simulink model "Ver1"  (R2025a)
settings: Solver=VariableStepAuto  StartTime=0.0  StopTime=50  RelTol=1e-3
model workspace (MAT data in the model file):
  params = Simulink.Parameter
  params.Value.graph_params.n_drones = 10
  params.Value.graph_params.n_vertex = 10
  params.Value.graph_params.dim = 3
  params.Value.graph_params.edges = [1  2; 1  3; 1  4; 1  5; 1  6; 1  7; 1  8; 1  9; 1  10; 2  3; 3  4; 4  5; 5  6; 6  7; 7  8; 8  9; 9  10; 10  2; 2  4; 3  5; 4  6; 5  7; 6  8; 7  9; 8  10; 9  2; 2  5; 3  6; 4  7; 5  8; 6  9; 7  10; 8  2; 9  3; 2  7; 3  8; 4  9; 5  10]
  params.Value.leader_params.gamma_leader = 5
  params.Value.leader_params.beta_leader = 20
  params.Value.formation_params.alpha = 0.1
  params.Value.formation_params.beta = 5
  params.Value.formation_params.kp = 0.1
  params.Value.formation_params.kd = 0.2
  params.Value.formation_params.d_star = [12; 12.3583419921; 12.0437867802; 12.2780291578; 12.153953398; 12.153953398; 12.2780291578; 12.0437867802; 12.3583419921; 8.7239794346; 8.43195016483; 8.97293523752; 8.23575839836; 9.06937336224; 8.23575839836; 8.97293523752; 8.43195016483; 8.7239794346; 15.4609871883; 16.3957181972; 15.70725761; 16.0772502381; 16.0772502381; 15.70725761; 16.3957181972; 15.4609871883; 20.9463600657; 21.3504473017; 20.8041858677; 21.4242852856; 20.8041858677; 21.3504473017; 20.9463600657; 21.1623309302; 23.7139211854; 23.6380722142; 23.7243055707; 23.6380722142]
  params.Value.avoid_params.k = 0.3
  params.Value.avoid_params.alpha = 2
  params.Value.avoid_params.d_safe = 5
  params.Value.conn_params.omega = 30
  params.Value.conn_params.alpha = 4
  params.Value.conn_params.d_max = 100
  params.Value.conn_params.Q = [-0.504121366584  -0.26105915892  -0.171736950093  -0.315040358305  -0.405829965319  0.0998199433836  -0.438792761923  -0.20112384887  0.203258169728; 0.156957729109  -0.265892972159  -0.546045591004  0.250622322861  0.326889653272  0.0848989604996  -0.256821652418  -0.050927060205  -0.510952303973; -0.317453653204  -0.3194315981  0.431976209598  -0.0284937114609  0.594225330731  -0.201716490834  0.193668666917  -0.272418527482  0.0652579645217; -0.13048124049  -0.134179261876  0.122212763196  -0.0870348158074  -0.0371148175386  -0.151496335719  0.0161251708109  0.899410389048  -0.0945083828758; 0.192528892253  -0.114548534632  0.205433346657  -0.218675435515  -0.474708640435  0.0269386697665  0.459932147337  -0.227364089546  -0.52008024212; 0.369488953482  0.322391236465  0.52165561704  -0.0285219597056  0.0532846827894  0.159326821637  -0.592803250035  -0.0504485144303  -0.0664731491506; -0.415313062767  0.706628196345  -0.139244596418  0.283837891368  -0.0540882463489  -0.300425585948  0.0949860236049  -0.0883544592836  -0.135013775508; 0.450114303089  0.121748450665  -0.342077032843  -0.467416117234  0.120960097676  -0.427451020909  0.0961435138919  -0.0562630144241  0.370573991674; 0.231595539246  -0.260589900824  0.050268923297  0.689669598678  -0.307348035599  -0.0738893443802  0.0890571931834  -0.0373520916293  0.437077198207; -0.033316094133  0.204933543037  -0.132442689429  -0.0789474148786  0.183729940772  0.783994382503  0.338504948631  0.0848412168229  0.250860529497]
  params.Value.estimation_params.mu = 1.2
  params.Value.prior_params.k_form = 5
  params.Value.prior_params.k_back = 1
  params.Value.prior_params.k_damp = 1
  params.Value.prior_params.k_conn = 0.5
  params.Value.prior_params.k_avoid = 10
  params.Value.prior_params.k_height = 25
  params.Complexity = 'real'
  params.Dimensions = [1 1]
  params.DataType = 'Bus: slBus8'
values from neighbouring files (symbols this model uses):
  edges = getappdata(0, 'DataEdges')    [DataAnalysis.m]    (also in Data_Analysis.m = graph_params.edges; Trajectory.m = getappdata(0, 'Edges'); data.m = graph_params.edges; formation_data.mat = [1 1 1 1 1 1 1 1 1 1 2 3 ... (62 elements, 31x2)])
  p10_init = [9; 5; 0]    [data.m]
  p2_init = [10; 0; 0]    [data.m]
  p3_init = [0; 10; 0]    [data.m]
  p4_init = [-10; 0; 0]    [data.m]
  p5_init = [0; -10; 0]    [data.m]
  p6_init = [7; 7; 0]    [data.m]
  p7_init = [-7; 7; 0]    [data.m]
  p8_init = [-7; -7; 0]    [data.m]
  p9_init = [7; -7; 0]    [data.m]
(part 1 of 3)
settings Model: Creator=huy01  LastModifiedBy=huy01

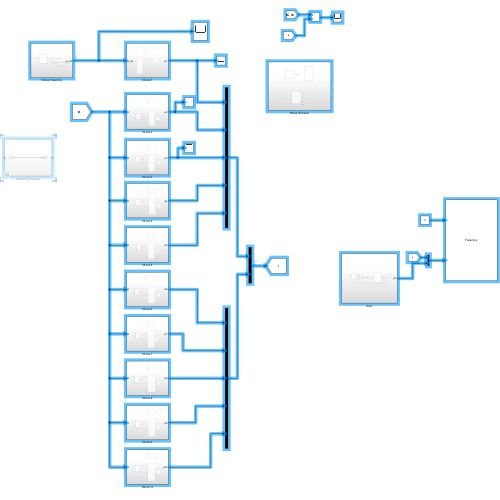
[thumbnail: Simulink's stored preview of the top-level diagram]
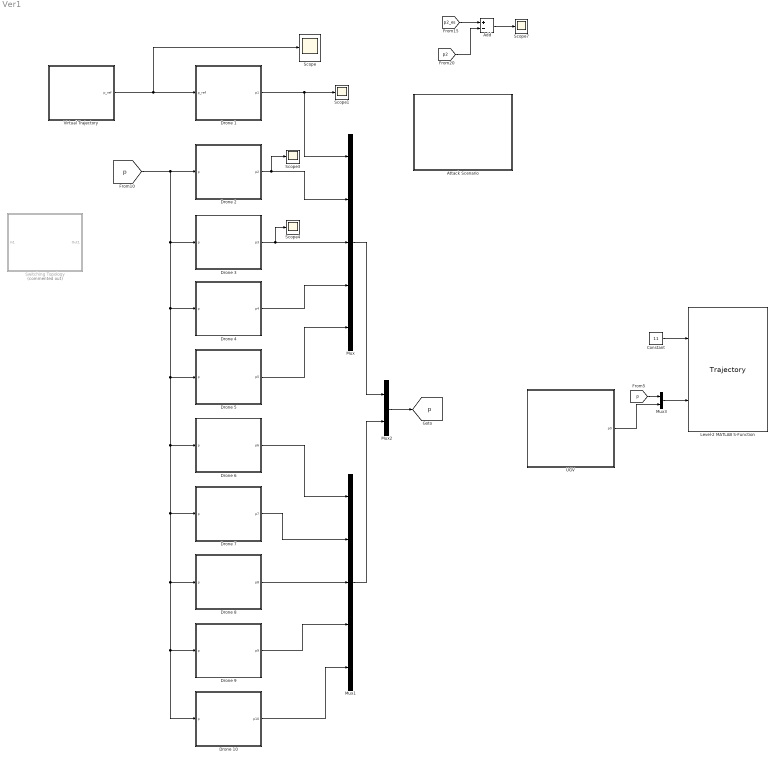
== system Ver1 ==
  Add : Sum  Inputs=+-
  Attack Scenario : Subsystem
  Constant : Constant  Value=11
  Drone 1 : Subsystem
  Drone 10 : Subsystem
  Drone 2 : Subsystem
  Drone 3 : Subsystem
  Drone 4 : Subsystem
  Drone 5 : Subsystem
  Drone 6 : Subsystem
  Drone 7 : Subsystem
  Drone 8 : Subsystem
  Drone 9 : Subsystem
  Level-2 MATLAB S-Function : M-S-Function  FunctionName=Trajectory
  Mux : Mux  Inputs=5
  Mux1 : Mux  Inputs=5
  Mux2 : Mux  Inputs=2
  Mux3 : Mux  Inputs=2
  Scope{,1,3..4,7} (5 alike) : Scope
      Scope settings: ActiveDisplayYMinimum=-6.2499999999999982  ActiveDisplayYMaximum=56.25
      Scope1 settings: ActiveDisplayYMinimum=-3.1816184672991272  ActiveDisplayYMaximum=28.634566205692153
      Scope3 settings: ActiveDisplayYMinimum=-20.171264012877725  ActiveDisplayYMaximum=51.444926631069329  DataLoggingVariableName=ScopeData3
      Scope4 settings: ActiveDisplayYMinimum=-35.468264300452987  ActiveDisplayYMaximum=33.637957066493193  DataLoggingVariableName=ScopeData4
      Scope7 settings: ActiveDisplayYMinimum=-11.251507111001377  ActiveDisplayYMaximum=1.2635639990123921  DataLoggingVariableName=ScopeData10
  Switching Topology : Subsystem  Commented=on
  UGV : Subsystem
  Virtual Trajectory : Subsystem
  tag scope: p=global
  wires:
  UGV/1(p0) -> Mux3/2
  [p2] -> Add/2
  Mux/1 -> Mux2/1
  Drone 10/1(p10) -> Mux1/5
  Mux3/1 -> Level-2 MATLAB S-Function/2
  [p] -> Mux3/1
  Drone 1/1(p1) -> Mux/1, Scope1/1
  [p2_es] -> Add/1
  [p] -> Drone 5/1(p), Drone 10/1(p), Drone 9/1(p), Drone 8/1(p), Drone 7/1(p), Drone 6/1(p), Drone 4/1(p), Drone 3/1(p), Drone 2/1(p)
  Add/1 -> Scope7/1
  Mux1/1 -> Mux2/2
  Drone 2/1(p2) -> Scope3/1, Mux/2
  Drone 9/1(p9) -> Mux1/4
  Drone 6/1(p6) -> Mux1/1
  Drone 5/1(p5) -> Mux/5
  Constant/1 -> Level-2 MATLAB S-Function/1
  Mux2/1 -> [p]
  Drone 4/1(p4) -> Mux/4
  Drone 7/1(p7) -> Mux1/2
  Drone 3/1(p3) -> Scope4/1, Mux/3
  Drone 8/1(p8) -> Mux1/3
  Virtual Trajectory/1(p_ref) -> Scope/1, Drone 1/1(p_ref)

== system Ver1/Attack Scenario ==
  Attacker : MATLAB Function  Commented=on  TreatAsAtomicUnit=on
  Data : Subsystem
  MATLAB Function : MATLAB Function  TreatAsAtomicUnit=on
  Scope : Scope
      settings: ActiveDisplayYMinimum=-20.35285300251708  ActiveDisplayYMaximum=217.26420858699828  DataLoggingVariableName=ScopeData2
  Scope1 : Scope
      settings: ActiveDisplayYMinimum=3.25  ActiveDisplayYMaximum=10.75  DataLoggingVariableName=ScopeData5
  Scope2 : Scope
      settings: ActiveDisplayYMinimum=-1.2499999999999998  ActiveDisplayYMaximum=11.25  DataLoggingVariableName=ScopeData6
  tag scope: n=global, p_es=global
  wires:
  Data/1(pes) -> [p_es]
  [p] -> MATLAB Function/1(p)
  [p0] -> MATLAB Function/2(p0)
  MATLAB Function/1(d1) -> Scope/1
  MATLAB Function/2(i_min) -> Scope1/1
  MATLAB Function/3(n) -> [n], Scope2/1

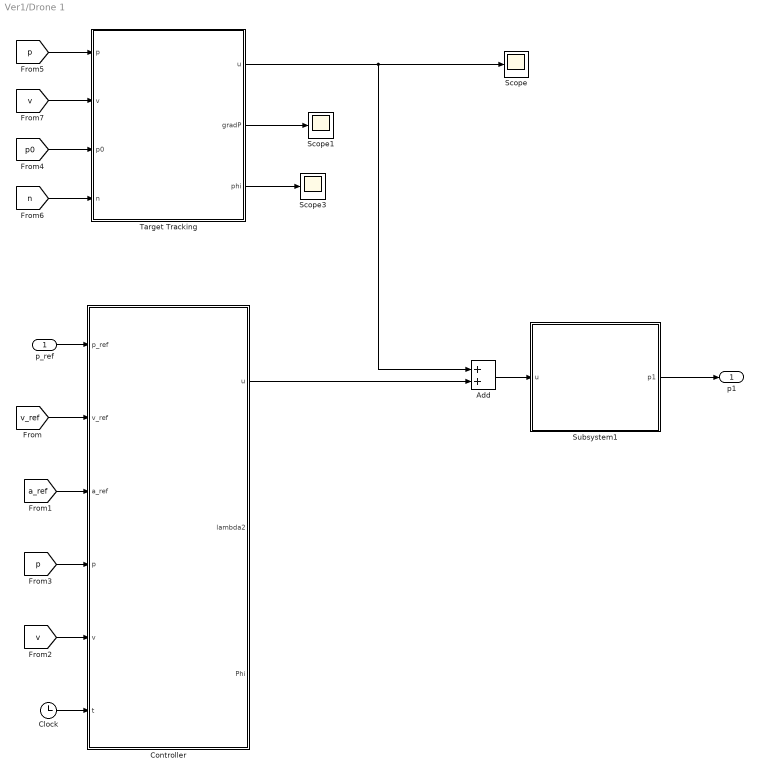
== system Ver1/Drone 1 ==
  p_ref : Inport
  Add : Sum
  Clock : Clock
  Controller : MATLAB Function  TreatAsAtomicUnit=on
  Scope : Scope
      settings: ActiveDisplayYMinimum=-25  ActiveDisplayYMaximum=25  DataLoggingVariableName=ScopeData17
  Scope1 : Scope
      settings: ActiveDisplayYMinimum=-1  ActiveDisplayYMaximum=1  DataLoggingVariableName=ScopeData18
  Scope3 : Scope
      settings: ActiveDisplayYMinimum=-1.1694156754654319E+234  ActiveDisplayYMaximum=1.0524741079188889E+235  DataLoggingVariableName=ScopeData20
  Subsystem1 : Subsystem
  Target Tracking : MATLAB Function  TreatAsAtomicUnit=on
  p1 : Outport
  wires:
  [v] -> Controller/5(v)
  [p] -> Controller/4(p)
  Subsystem1/1(p1) -> p1/1
  [p0] -> Target Tracking/3(p0)
  [p] -> Target Tracking/1(p)
  Target Tracking/1(u) -> Scope/1, Add/1
  [n] -> Target Tracking/4(n)
  Target Tracking/2(gradP) -> Scope1/1
  [v] -> Target Tracking/2(v)
  Target Tracking/3(phi) -> Scope3/1
  Add/1 -> Subsystem1/1(u)
  Controller/1(u) -> Add/2
  p_ref/1 -> Controller/1(p_ref)
  [a_ref] -> Controller/3(a_ref)
  Clock/1 -> Controller/6(t)
  [v_ref] -> Controller/2(v_ref)

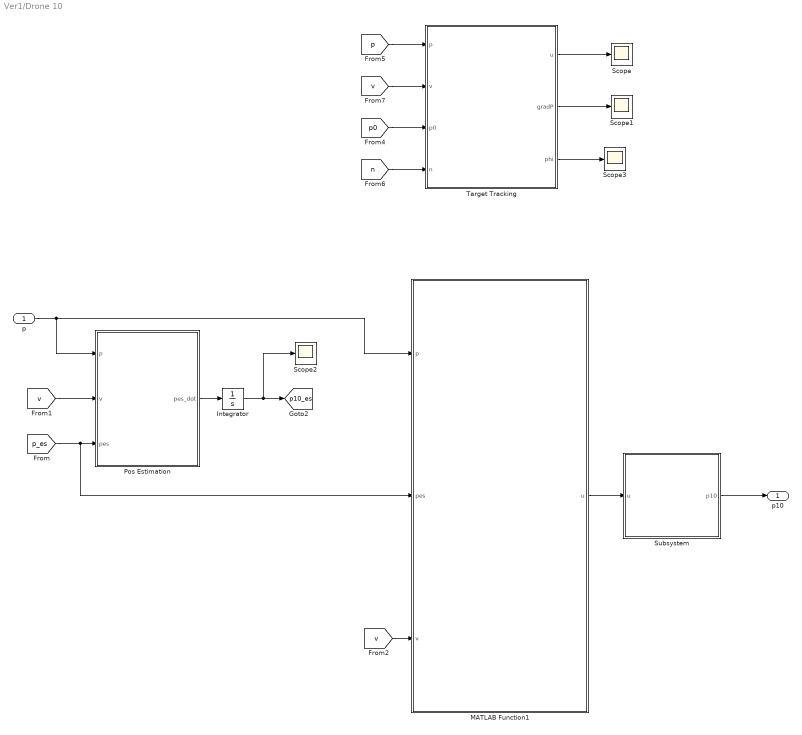
== system Ver1/Drone 10 ==
  p : Inport
  Integrator : Integrator  InitialCondition=[0;0;0]
  MATLAB Function1 : MATLAB Function  TreatAsAtomicUnit=on
  Pos Estimation : MATLAB Function  TreatAsAtomicUnit=on
  Scope{,1..3} (4 alike) : Scope
      Scope settings: ActiveDisplayYMinimum=-25  ActiveDisplayYMaximum=25  DataLoggingVariableName=ScopeData44
      Scope1 settings: ActiveDisplayYMinimum=-1  ActiveDisplayYMaximum=1  DataLoggingVariableName=ScopeData45
      Scope2 settings: DataLoggingVariableName=ScopeData13
      Scope3 settings: ActiveDisplayYMinimum=-1.1694156754654319E+234  ActiveDisplayYMaximum=1.0524741079188889E+235  DataLoggingVariableName=ScopeData46
  Subsystem : Subsystem
  Target Tracking : MATLAB Function  TreatAsAtomicUnit=on
  p10 : Outport
  tag scope: p10_es=global
  wires:
  Subsystem/1(p10) -> p10/1
  [v] -> MATLAB Function1/3(v)
  Integrator/1 -> Scope2/1, [p10_es]
  p/1 -> Pos Estimation/1(p), MATLAB Function1/1(p)
  Pos Estimation/1(pes_dot) -> Integrator/1
  [p_es] -> MATLAB Function1/2(pes), Pos Estimation/3(pes)
  [v] -> Target Tracking/2(v)
  Target Tracking/3(phi) -> Scope3/1
  [p0] -> Target Tracking/3(p0)
  Target Tracking/2(gradP) -> Scope1/1
  [n] -> Target Tracking/4(n)
  Target Tracking/1(u) -> Scope/1
  [p] -> Target Tracking/1(p)
  MATLAB Function1/1(u) -> Subsystem/1(u)
  [v] -> Pos Estimation/2(v)

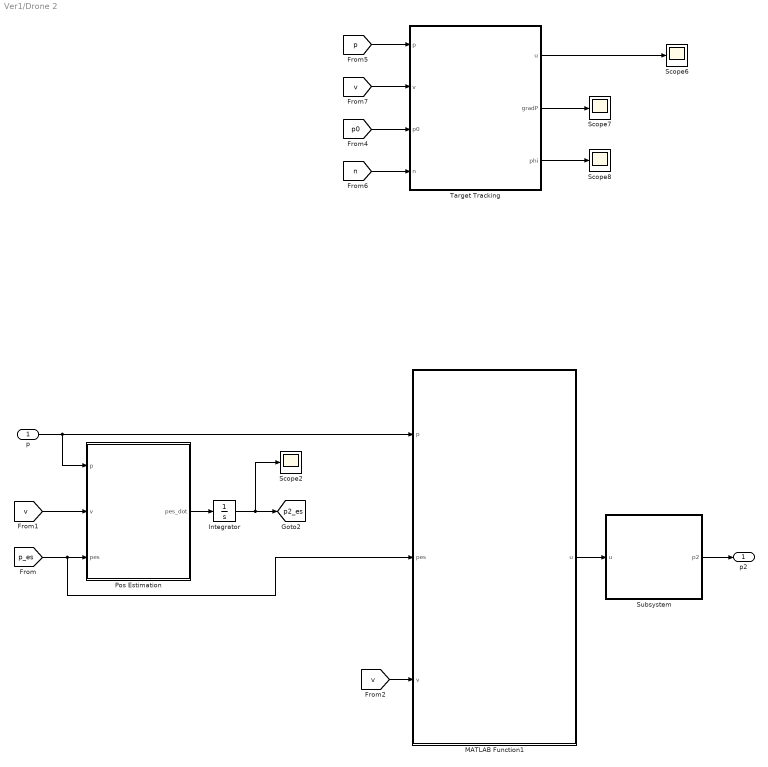
== system Ver1/Drone 2 ==
  p : Inport
  Integrator : Integrator  InitialCondition=[0;0;0]
  MATLAB Function1 : MATLAB Function  TreatAsAtomicUnit=on
  Pos Estimation : MATLAB Function  TreatAsAtomicUnit=on
  Scope{2,6..8} (4 alike) : Scope
      Scope2 settings: ActiveDisplayYMinimum=-1  ActiveDisplayYMaximum=1  DataLoggingVariableName=ScopeData9
      Scope6 settings: ActiveDisplayYMinimum=-25  ActiveDisplayYMaximum=25  DataLoggingVariableName=ScopeData19
      Scope7 settings: ActiveDisplayYMinimum=-1  ActiveDisplayYMaximum=1  DataLoggingVariableName=ScopeData21
      Scope8 settings: ActiveDisplayYMinimum=-1.1694156754654319E+234  ActiveDisplayYMaximum=1.0524741079188889E+235  DataLoggingVariableName=ScopeData22
  Subsystem : Subsystem
  Target Tracking : MATLAB Function  TreatAsAtomicUnit=on
  p2 : Outport
  tag scope: p2_es=global
  wires:
  [v] -> MATLAB Function1/3(v)
  p/1 -> Pos Estimation/1(p), MATLAB Function1/1(p)
  Subsystem/1(p2) -> p2/1
  Pos Estimation/1(pes_dot) -> Integrator/1
  Integrator/1 -> Scope2/1, [p2_es]
  [p_es] -> MATLAB Function1/2(pes), Pos Estimation/3(pes)
  [v] -> Target Tracking/2(v)
  Target Tracking/3(phi) -> Scope8/1
  [p0] -> Target Tracking/3(p0)
  Target Tracking/2(gradP) -> Scope7/1
  [n] -> Target Tracking/4(n)
  Target Tracking/1(u) -> Scope6/1
  [p] -> Target Tracking/1(p)
  MATLAB Function1/1(u) -> Subsystem/1(u)
  [v] -> Pos Estimation/2(v)

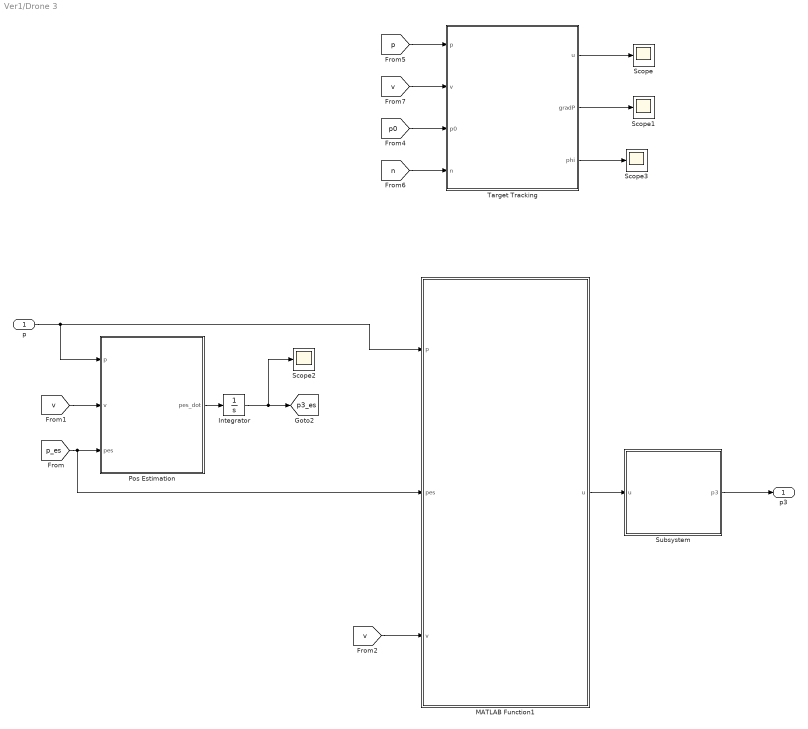
== system Ver1/Drone 3 ==
  p : Inport
  Integrator : Integrator  InitialCondition=[0;0;0]
  MATLAB Function1 : MATLAB Function  TreatAsAtomicUnit=on
  Pos Estimation : MATLAB Function  TreatAsAtomicUnit=on
  Scope{,1..3} (4 alike) : Scope
      Scope settings: ActiveDisplayYMinimum=-25  ActiveDisplayYMaximum=25  DataLoggingVariableName=ScopeData23
      Scope1 settings: ActiveDisplayYMinimum=-1  ActiveDisplayYMaximum=1  DataLoggingVariableName=ScopeData24
      Scope2 settings: ActiveDisplayYMinimum=-1  ActiveDisplayYMaximum=1  DataLoggingVariableName=ScopeData11
      Scope3 settings: ActiveDisplayYMinimum=-1.1694156754654319E+234  ActiveDisplayYMaximum=1.0524741079188889E+235  DataLoggingVariableName=ScopeData25
  Subsystem : Subsystem
  Target Tracking : MATLAB Function  TreatAsAtomicUnit=on
  p3 : Outport
  tag scope: p3_es=global
  wires:
  Subsystem/1(p3) -> p3/1
  [v] -> MATLAB Function1/3(v)
  Integrator/1 -> Scope2/1, [p3_es]
  p/1 -> Pos Estimation/1(p), MATLAB Function1/1(p)
  Pos Estimation/1(pes_dot) -> Integrator/1
  [p_es] -> MATLAB Function1/2(pes), Pos Estimation/3(pes)
  [v] -> Target Tracking/2(v)
  Target Tracking/3(phi) -> Scope3/1
  [p0] -> Target Tracking/3(p0)
  Target Tracking/2(gradP) -> Scope1/1
  [n] -> Target Tracking/4(n)
  Target Tracking/1(u) -> Scope/1
  [p] -> Target Tracking/1(p)
  MATLAB Function1/1(u) -> Subsystem/1(u)
  [v] -> Pos Estimation/2(v)

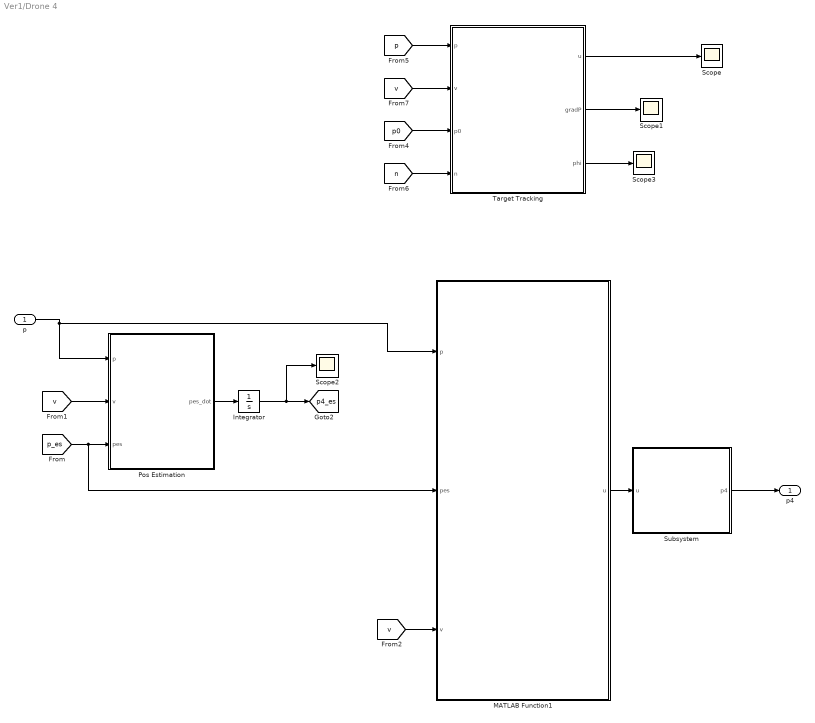
== system Ver1/Drone 4 ==
  p : Inport
  Integrator : Integrator  InitialCondition=[0;0;0]
  MATLAB Function1 : MATLAB Function  TreatAsAtomicUnit=on
  Pos Estimation : MATLAB Function  TreatAsAtomicUnit=on
  Scope{,1..3} (4 alike) : Scope
      Scope settings: ActiveDisplayYMinimum=-25  ActiveDisplayYMaximum=25  DataLoggingVariableName=ScopeData26
      Scope1 settings: ActiveDisplayYMinimum=-1  ActiveDisplayYMaximum=1  DataLoggingVariableName=ScopeData27
      Scope2 settings: DataLoggingVariableName=ScopeData12
      Scope3 settings: ActiveDisplayYMinimum=-1.1694156754654319E+234  ActiveDisplayYMaximum=1.0524741079188889E+235  DataLoggingVariableName=ScopeData28
  Subsystem : Subsystem
  Target Tracking : MATLAB Function  TreatAsAtomicUnit=on
  p4 : Outport
  tag scope: p4_es=global
  wires:
  Subsystem/1(p4) -> p4/1
  [v] -> MATLAB Function1/3(v)
  Integrator/1 -> Scope2/1, [p4_es]
  p/1 -> Pos Estimation/1(p), MATLAB Function1/1(p)
  Pos Estimation/1(pes_dot) -> Integrator/1
  [p_es] -> MATLAB Function1/2(pes), Pos Estimation/3(pes)
  [v] -> Target Tracking/2(v)
  Target Tracking/3(phi) -> Scope3/1
  [p0] -> Target Tracking/3(p0)
  Target Tracking/2(gradP) -> Scope1/1
  [n] -> Target Tracking/4(n)
  Target Tracking/1(u) -> Scope/1
  [p] -> Target Tracking/1(p)
  MATLAB Function1/1(u) -> Subsystem/1(u)
  [v] -> Pos Estimation/2(v)

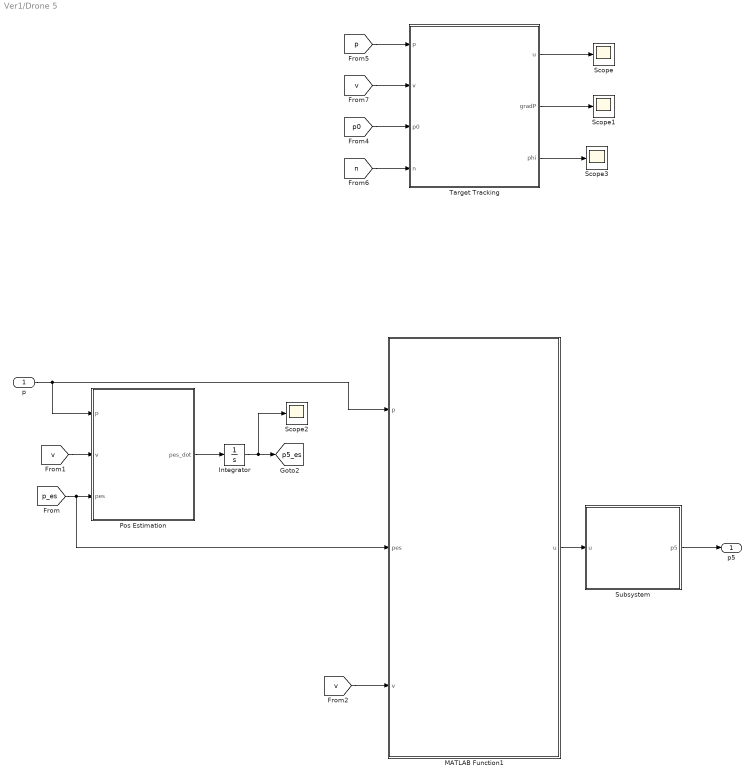
== system Ver1/Drone 5 ==
  p : Inport
  Integrator : Integrator  InitialCondition=[0;0;0]
  MATLAB Function1 : MATLAB Function  TreatAsAtomicUnit=on
  Pos Estimation : MATLAB Function  TreatAsAtomicUnit=on
  Scope{,1..3} (4 alike) : Scope
      Scope settings: ActiveDisplayYMinimum=-25  ActiveDisplayYMaximum=25  DataLoggingVariableName=ScopeData29
      Scope1 settings: ActiveDisplayYMinimum=-1  ActiveDisplayYMaximum=1  DataLoggingVariableName=ScopeData30
      Scope2 settings: DataLoggingVariableName=ScopeData13
      Scope3 settings: ActiveDisplayYMinimum=-1.1694156754654319E+234  ActiveDisplayYMaximum=1.0524741079188889E+235  DataLoggingVariableName=ScopeData31
  Subsystem : Subsystem
  Target Tracking : MATLAB Function  TreatAsAtomicUnit=on
  p5 : Outport
  tag scope: p5_es=global
  wires:
  Subsystem/1(p5) -> p5/1
  [v] -> MATLAB Function1/3(v)
  Integrator/1 -> Scope2/1, [p5_es]
  p/1 -> Pos Estimation/1(p), MATLAB Function1/1(p)
  Pos Estimation/1(pes_dot) -> Integrator/1
  [p_es] -> MATLAB Function1/2(pes), Pos Estimation/3(pes)
  [v] -> Target Tracking/2(v)
  Target Tracking/3(phi) -> Scope3/1
  [p0] -> Target Tracking/3(p0)
  Target Tracking/2(gradP) -> Scope1/1
  [n] -> Target Tracking/4(n)
  Target Tracking/1(u) -> Scope/1
  [p] -> Target Tracking/1(p)
  MATLAB Function1/1(u) -> Subsystem/1(u)
  [v] -> Pos Estimation/2(v)
  ? -> ?

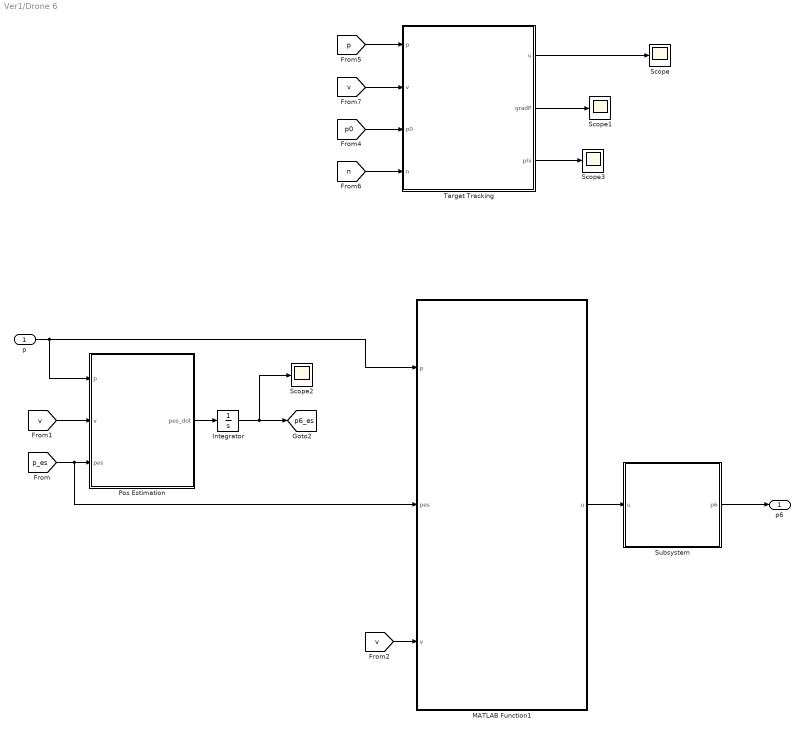
== system Ver1/Drone 6 ==
  p : Inport
  Integrator : Integrator  InitialCondition=[0;0;0]
  MATLAB Function1 : MATLAB Function  TreatAsAtomicUnit=on
  Pos Estimation : MATLAB Function  TreatAsAtomicUnit=on
  Scope{,1..3} (4 alike) : Scope
      Scope settings: ActiveDisplayYMinimum=-25  ActiveDisplayYMaximum=25  DataLoggingVariableName=ScopeData32
      Scope1 settings: ActiveDisplayYMinimum=-1  ActiveDisplayYMaximum=1  DataLoggingVariableName=ScopeData33
      Scope2 settings: DataLoggingVariableName=ScopeData13
      Scope3 settings: ActiveDisplayYMinimum=-1.1694156754654319E+234  ActiveDisplayYMaximum=1.0524741079188889E+235  DataLoggingVariableName=ScopeData34
  Subsystem : Subsystem
  Target Tracking : MATLAB Function  TreatAsAtomicUnit=on
  p6 : Outport
  tag scope: p6_es=global
  wires:
  Subsystem/1(p6) -> p6/1
  [v] -> MATLAB Function1/3(v)
  Integrator/1 -> Scope2/1, [p6_es]
  p/1 -> Pos Estimation/1(p), MATLAB Function1/1(p)
  Pos Estimation/1(pes_dot) -> Integrator/1
  [p_es] -> MATLAB Function1/2(pes), Pos Estimation/3(pes)
  [v] -> Target Tracking/2(v)
  Target Tracking/3(phi) -> Scope3/1
  [p0] -> Target Tracking/3(p0)
  Target Tracking/2(gradP) -> Scope1/1
  [n] -> Target Tracking/4(n)
  Target Tracking/1(u) -> Scope/1
  [p] -> Target Tracking/1(p)
  MATLAB Function1/1(u) -> Subsystem/1(u)
  [v] -> Pos Estimation/2(v)

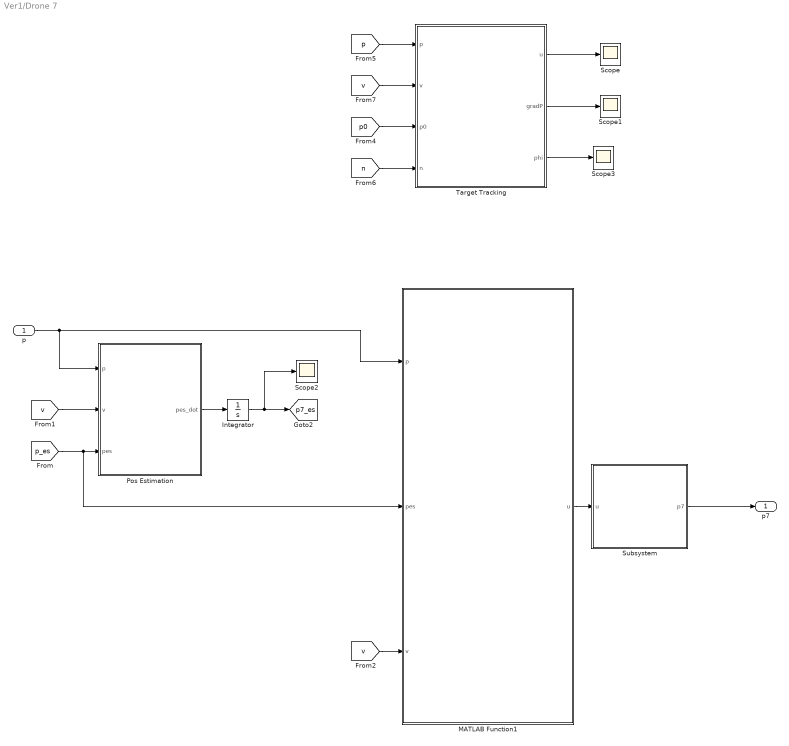
== system Ver1/Drone 7 ==
  p : Inport
  Integrator : Integrator  InitialCondition=[0;0;0]
  MATLAB Function1 : MATLAB Function  TreatAsAtomicUnit=on
  Pos Estimation : MATLAB Function  TreatAsAtomicUnit=on
  Scope{,1..3} (4 alike) : Scope
      Scope settings: ActiveDisplayYMinimum=-25  ActiveDisplayYMaximum=25  DataLoggingVariableName=ScopeData35
      Scope1 settings: ActiveDisplayYMinimum=-1  ActiveDisplayYMaximum=1  DataLoggingVariableName=ScopeData36
      Scope2 settings: DataLoggingVariableName=ScopeData13
      Scope3 settings: ActiveDisplayYMinimum=-1.1694156754654319E+234  ActiveDisplayYMaximum=1.0524741079188889E+235  DataLoggingVariableName=ScopeData37
  Subsystem : Subsystem
  Target Tracking : MATLAB Function  TreatAsAtomicUnit=on
  p7 : Outport
  tag scope: p7_es=global
  wires:
  Subsystem/1(p7) -> p7/1
  [v] -> MATLAB Function1/3(v)
  Integrator/1 -> Scope2/1, [p7_es]
  p/1 -> Pos Estimation/1(p), MATLAB Function1/1(p)
  Pos Estimation/1(pes_dot) -> Integrator/1
  [p_es] -> MATLAB Function1/2(pes), Pos Estimation/3(pes)
  [v] -> Target Tracking/2(v)
  Target Tracking/3(phi) -> Scope3/1
  [p0] -> Target Tracking/3(p0)
  Target Tracking/2(gradP) -> Scope1/1
  [n] -> Target Tracking/4(n)
  Target Tracking/1(u) -> Scope/1
  [p] -> Target Tracking/1(p)
  MATLAB Function1/1(u) -> Subsystem/1(u)
  [v] -> Pos Estimation/2(v)

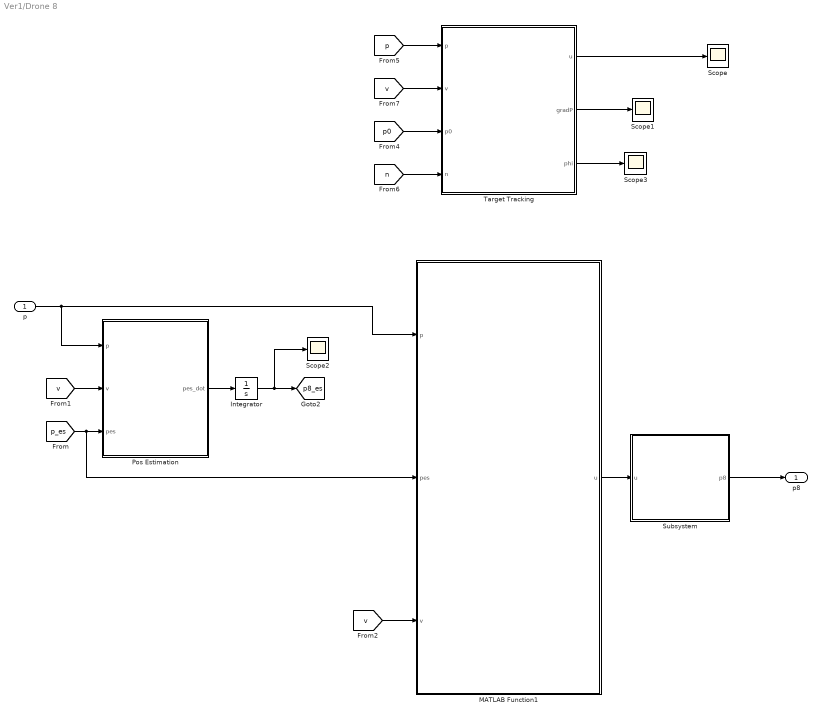
== system Ver1/Drone 8 ==
  p : Inport
  Integrator : Integrator  InitialCondition=[0;0;0]
  MATLAB Function1 : MATLAB Function  TreatAsAtomicUnit=on
  Pos Estimation : MATLAB Function  TreatAsAtomicUnit=on
  Scope{,1..3} (4 alike) : Scope
      Scope settings: ActiveDisplayYMinimum=-25  ActiveDisplayYMaximum=25  DataLoggingVariableName=ScopeData38
      Scope1 settings: ActiveDisplayYMinimum=-1  ActiveDisplayYMaximum=1  DataLoggingVariableName=ScopeData39
      Scope2 settings: DataLoggingVariableName=ScopeData13
      Scope3 settings: ActiveDisplayYMinimum=-1.1694156754654319E+234  ActiveDisplayYMaximum=1.0524741079188889E+235  DataLoggingVariableName=ScopeData40
  Subsystem : Subsystem
  Target Tracking : MATLAB Function  TreatAsAtomicUnit=on
  p8 : Outport
  tag scope: p8_es=global
  wires:
  Subsystem/1(p8) -> p8/1
  [v] -> MATLAB Function1/3(v)
  Integrator/1 -> Scope2/1, [p8_es]
  p/1 -> Pos Estimation/1(p), MATLAB Function1/1(p)
  Pos Estimation/1(pes_dot) -> Integrator/1
  [p_es] -> MATLAB Function1/2(pes), Pos Estimation/3(pes)
  [v] -> Target Tracking/2(v)
  Target Tracking/3(phi) -> Scope3/1
  [p0] -> Target Tracking/3(p0)
  Target Tracking/2(gradP) -> Scope1/1
  [n] -> Target Tracking/4(n)
  Target Tracking/1(u) -> Scope/1
  [p] -> Target Tracking/1(p)
  [v] -> Pos Estimation/2(v)
  MATLAB Function1/1(u) -> Subsystem/1(u)

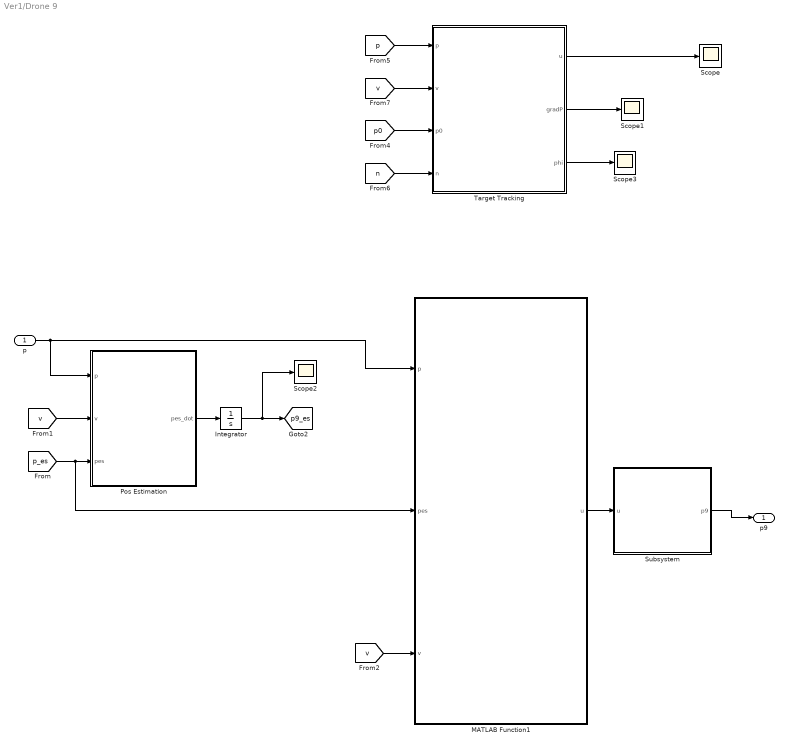
== system Ver1/Drone 9 ==
  p : Inport
  Integrator : Integrator  InitialCondition=[0;0;0]
  MATLAB Function1 : MATLAB Function  TreatAsAtomicUnit=on
  Pos Estimation : MATLAB Function  TreatAsAtomicUnit=on
  Scope{,1..3} (4 alike) : Scope
      Scope settings: ActiveDisplayYMinimum=-25  ActiveDisplayYMaximum=25  DataLoggingVariableName=ScopeData41
      Scope1 settings: ActiveDisplayYMinimum=-1  ActiveDisplayYMaximum=1  DataLoggingVariableName=ScopeData42
      Scope2 settings: DataLoggingVariableName=ScopeData13
      Scope3 settings: ActiveDisplayYMinimum=-1.1694156754654319E+234  ActiveDisplayYMaximum=1.0524741079188889E+235  DataLoggingVariableName=ScopeData43
  Subsystem : Subsystem
  Target Tracking : MATLAB Function  TreatAsAtomicUnit=on
  p9 : Outport
  tag scope: p9_es=global
  wires:
  Subsystem/1(p9) -> p9/1
  [v] -> MATLAB Function1/3(v)
  Integrator/1 -> Scope2/1, [p9_es]
  p/1 -> Pos Estimation/1(p), MATLAB Function1/1(p)
  Pos Estimation/1(pes_dot) -> Integrator/1
  [p_es] -> MATLAB Function1/2(pes), Pos Estimation/3(pes)
  [v] -> Target Tracking/2(v)
  Target Tracking/3(phi) -> Scope3/1
  [p0] -> Target Tracking/3(p0)
  Target Tracking/2(gradP) -> Scope1/1
  [n] -> Target Tracking/4(n)
  Target Tracking/1(u) -> Scope/1
  [p] -> Target Tracking/1(p)
  MATLAB Function1/1(u) -> Subsystem/1(u)
  [v] -> Pos Estimation/2(v)

== system Ver1/Switching Topology ==
  In1 : Inport
  Out1 : Outport
  wires:
  In1/1 -> Out1/1

== system Ver1/UGV ==
  Add : Sum  Inputs=+-
  Clock : Clock
  Constant : Constant  Value=0
  Gain : Gain  Gain=10
  Integrator : Integrator  InitialCondition=zeros(3,1)
  MATLAB Function : MATLAB Function  TreatAsAtomicUnit=on
  MATLAB Function1 : MATLAB Function  TreatAsAtomicUnit=on
  Mux : Mux  Inputs=2
  p0 : Outport
  tag scope: p0=global
  wires:
  MATLAB Function/1(psi_dot) -> Integrator/1
  Integrator/1 -> [p0], Add/2, p0/1
  MATLAB Function1/1(psi_ref) -> Mux/1
  Constant/1 -> Mux/2
  Mux/1 -> Add/1
  Add/1 -> Gain/1
  Gain/1 -> MATLAB Function/1(u)
  Clock/1 -> MATLAB Function1/1(t)

== system Ver1/Virtual Trajectory ==
  Clock : Clock
  Derivative : Derivative
  Derivative1 : Derivative
  MATLAB Function : MATLAB Function  TreatAsAtomicUnit=on
  p_ref : Outport
  tag scope: a_ref=global, v_ref=global
  wires:
  MATLAB Function/1(p_ref) -> Derivative/1, p_ref/1
  Clock/1 -> MATLAB Function/1(t)
  Derivative/1 -> Derivative1/1, [v_ref]
  Derivative1/1 -> [a_ref]

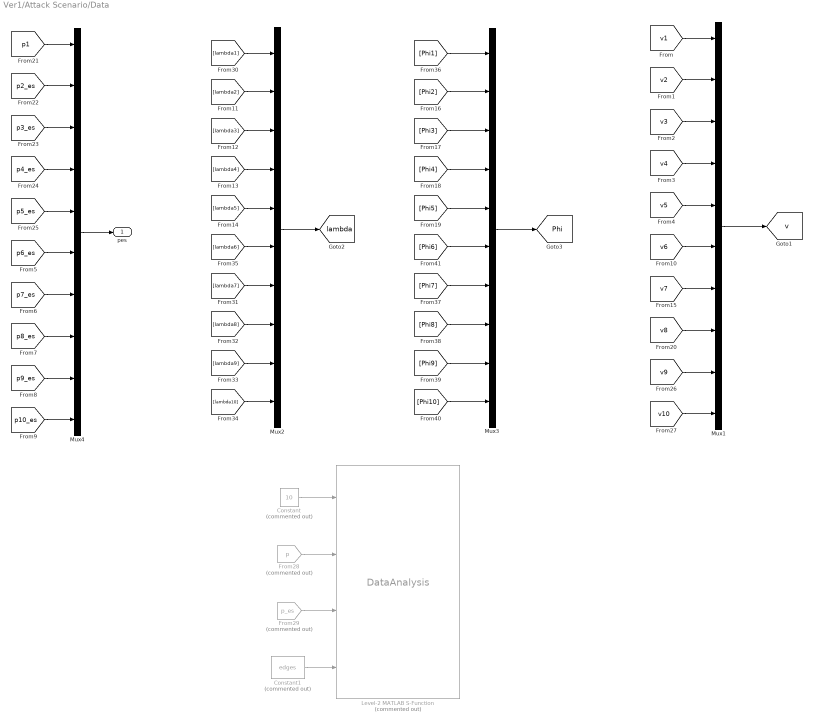
== system Ver1/Attack Scenario/Data ==
  Constant : Constant  Commented=on  Value=10
  Constant1 : Constant  Commented=on  Value=edges  VectorParams1D=off
  From28 : From  Commented=on  GotoTag=p  TagVisibility=global
  From29 : From  Commented=on  GotoTag=p_es  TagVisibility=global
  Level-2 MATLAB S-Function : M-S-Function  Commented=on  FunctionName=DataAnalysis
  Mux{1..4} (4 alike) : Mux  Inputs=10
  pes : Outport
  tag scope: Phi=global, lambda=global, v=global
  wires:
  [p2_es] -> Mux4/2
  [p4_es] -> Mux4/4
  [p3_es] -> Mux4/3
  [p5_es] -> Mux4/5
  [p1] -> Mux4/1
  [p6_es] -> Mux4/6
  [p7_es] -> Mux4/7
  [p8_es] -> Mux4/8
  [p9_es] -> Mux4/9
  [p10_es] -> Mux4/10
  [v1] -> Mux1/1
  [v2] -> Mux1/2
  [v3] -> Mux1/3
  [v4] -> Mux1/4
  [v5] -> Mux1/5
  [v6] -> Mux1/6
  [v7] -> Mux1/7
  [v8] -> Mux1/8
  [v9] -> Mux1/9
  [v10] -> Mux1/10
  Constant/1 -> Level-2 MATLAB S-Function/1
  From28/1 -> Level-2 MATLAB S-Function/2
  From29/1 -> Level-2 MATLAB S-Function/3
  Constant1/1 -> Level-2 MATLAB S-Function/4
  [lambda2] -> Mux2/2
  [lambda3] -> Mux2/3
  [lambda4] -> Mux2/4
  [lambda5] -> Mux2/5
  [lambda1] -> Mux2/1
  [lambda7] -> Mux2/7
  [lambda8] -> Mux2/8
  [lambda9] -> Mux2/9
  [lambda10] -> Mux2/10
  [lambda6] -> Mux2/6
  [Phi2] -> Mux3/2
  [Phi3] -> Mux3/3
  [Phi4] -> Mux3/4
  [Phi5] -> Mux3/5
  [Phi1] -> Mux3/1
  [Phi7] -> Mux3/7
  [Phi6] -> Mux3/6
  [Phi9] -> Mux3/9
  [Phi10] -> Mux3/10
  [Phi8] -> Mux3/8
  Mux4/1 -> pes/1
  Mux2/1 -> [lambda]
  Mux3/1 -> [Phi]
  Mux1/1 -> [v]

== system Ver1/Drone 1/Subsystem1 ==
  u : Inport
  Integrator : Integrator  InitialCondition=zeros(3,1)
  Integrator1 : Integrator  InitialCondition=[4;5;0];
  Kinematic : MATLAB Function  TreatAsAtomicUnit=on
  p1 : Outport
  tag scope: p1=global, v1=global
  wires:
  Integrator1/1 -> [p1], p1/1
  u/1 -> Kinematic/1(u)
  Integrator/1 -> [v1], Integrator1/1
  Kinematic/1(p_ddot) -> Integrator/1

== system Ver1/Drone 10/Subsystem ==
  u : Inport
  Integrator : Integrator  InitialCondition=zeros(3,1)
  Integrator1 : Integrator  InitialCondition=p10_init
  Kinematic : MATLAB Function  TreatAsAtomicUnit=on
  p10 : Outport
  tag scope: p10=global, v10=global
  wires:
  Integrator/1 -> [v10], Integrator1/1
  Integrator1/1 -> [p10], p10/1
  u/1 -> Kinematic/1(u)
  Kinematic/1(p_ddot) -> Integrator/1

== system Ver1/Drone 2/Subsystem ==
  u : Inport
  Integrator : Integrator  InitialCondition=zeros(3,1)
  Integrator1 : Integrator  InitialCondition=p2_init
  Kinematic : MATLAB Function  TreatAsAtomicUnit=on
  p2 : Outport
  tag scope: a2=global, p2=global, v2=global
  wires:
  Integrator/1 -> [v2], Integrator1/1
  Integrator1/1 -> [p2], p2/1
  u/1 -> Kinematic/1(u)
  Kinematic/1(p_ddot) -> [a2], Integrator/1

== system Ver1/Drone 3/Subsystem ==
  u : Inport
  Integrator : Integrator  InitialCondition=zeros(3,1)
  Integrator1 : Integrator  InitialCondition=p3_init
  Kinematic : MATLAB Function  TreatAsAtomicUnit=on
  p3 : Outport
  tag scope: p3=global, v3=global
  wires:
  Integrator/1 -> [v3], Integrator1/1
  Integrator1/1 -> [p3], p3/1
  u/1 -> Kinematic/1(u)
  Kinematic/1(p_ddot) -> Integrator/1

== system Ver1/Drone 4/Subsystem ==
  u : Inport
  Integrator : Integrator  InitialCondition=zeros(3,1)
  Integrator1 : Integrator  InitialCondition=p4_init
  Kinematic : MATLAB Function  TreatAsAtomicUnit=on
  p4 : Outport
  tag scope: p4=global, v4=global
  wires:
  Integrator/1 -> [v4], Integrator1/1
  Integrator1/1 -> [p4], p4/1
  u/1 -> Kinematic/1(u)
  Kinematic/1(p_ddot) -> Integrator/1

== system Ver1/Drone 5/Subsystem ==
  u : Inport
  Integrator : Integrator  InitialCondition=zeros(3,1)
  Integrator1 : Integrator  InitialCondition=p5_init
  Kinematic : MATLAB Function  TreatAsAtomicUnit=on
  p5 : Outport
  tag scope: p5=global, v5=global
  wires:
  Integrator/1 -> [v5], Integrator1/1
  Integrator1/1 -> [p5], p5/1
  u/1 -> Kinematic/1(u)
  Kinematic/1(p_ddot) -> Integrator/1

== system Ver1/Drone 6/Subsystem ==
  u : Inport
  Integrator : Integrator  InitialCondition=zeros(3,1)
  Integrator1 : Integrator  InitialCondition=p6_init
  Kinematic : MATLAB Function  TreatAsAtomicUnit=on
  p6 : Outport
  tag scope: p6=global, v6=global
  wires:
  Integrator/1 -> [v6], Integrator1/1
  Integrator1/1 -> [p6], p6/1
  u/1 -> Kinematic/1(u)
  Kinematic/1(p_ddot) -> Integrator/1

== system Ver1/Drone 7/Subsystem ==
  u : Inport
  Integrator : Integrator  InitialCondition=zeros(3,1)
  Integrator1 : Integrator  InitialCondition=p7_init
  Kinematic : MATLAB Function  TreatAsAtomicUnit=on
  p7 : Outport
  tag scope: p7=global, v7=global
  wires:
  Integrator/1 -> [v7], Integrator1/1
  Integrator1/1 -> [p7], p7/1
  u/1 -> Kinematic/1(u)
  Kinematic/1(p_ddot) -> Integrator/1

== system Ver1/Drone 8/Subsystem ==
  u : Inport
  Integrator : Integrator  InitialCondition=zeros(3,1)
  Integrator1 : Integrator  InitialCondition=p8_init
  Kinematic : MATLAB Function  TreatAsAtomicUnit=on
  p8 : Outport
  tag scope: p8=global, v8=global
  wires:
  Integrator/1 -> [v8], Integrator1/1
  Integrator1/1 -> [p8], p8/1
  u/1 -> Kinematic/1(u)
  Kinematic/1(p_ddot) -> Integrator/1

== system Ver1/Drone 9/Subsystem ==
  u : Inport
  Integrator : Integrator  InitialCondition=zeros(3,1)
  Integrator1 : Integrator  InitialCondition=p9_init
  Kinematic : MATLAB Function  TreatAsAtomicUnit=on
  p9 : Outport
  tag scope: p9=global, v9=global
  wires:
  Integrator/1 -> [v9], Integrator1/1
  Integrator1/1 -> [p9], p9/1
  u/1 -> Kinematic/1(u)
  Kinematic/1(p_ddot) -> Integrator/1

== matlab function Ver1/Drone 3/MATLAB Function1 ==
  data: p input; pes input; v input; u output; params parameter Bus: params_bus
function u = fcn(p, pes, v, params)

    graph_params = params.graph_params;
    formation_params = params.formation_params;
    conn_params = params.conn_params;
    avoid_params = params.avoid_params;
    prior_params = params.prior_params;

    % Chuyển vector p thành mảng 3x5
    pos = reshape(p, 3, graph_params.n_drones);
    vel = reshape(v, 3, graph_params.n_drones);
    pes = reshape(pes, 3, graph_params.n_drones);
    
    n_edges = size(graph_params.edges, 1);
    

    i_drone = 3;
    
    % =====================================================================
    %  FORMATION CONTROL (Distance-based + Backstepping)
    % =====================================================================
    u_form = zeros(3,1);
    gradV = zeros(3,1);
    dgradV = zeros(3,1);
    
    for e = 1:n_edges
        if graph_params.edges(e,1) == i_drone
            j = graph_params.edges(e,2);
            p_ij = pos(:,j) - pos(:,i_drone);
            v_ij = vel(:,j) - vel(:,i_drone);
            dij = norm(p_ij);
            
            if dij > 1e-6
                e_ij = dij^2 - formation_params.d_star(e)^2;
                
                % Lực formation (gradient descent)
                u_form = u_form + formation_params.alpha * e_ij * p_ij;
                
                % Gradient V
                gradV = gradV + e_ij * p_ij;
                
                % Đạo hàm gradient V
                term = 2*(p_ij' * v_ij) * p_ij + e_ij * v_ij;
                dgradV = dgradV + term;
            end
            
        elseif graph_params.edges(e,2) == i_drone
            j = graph_params.edges(e,1);
            p_ij = pos(:,j) - pos(:,i_drone);
            v_ij = vel(:,j) - vel(:,i_drone);
            dij = norm(p_ij);
            
            if dij > 1e-6
                e_ij = dij^2 - formation_params.d_star(e)^2;
                
                u_form = u_form + formation_params.alpha * e_ij * p_ij;
                gradV = gradV + e_ij * p_ij;
                term = 2*(p_ij' * v_ij) * p_ij + e_ij * v_ij;
                dgradV = dgradV + term;
            end
        end
    end
    
    % Giới hạn gradient
    gradV = max(min(gradV, 15), -15);
    dgradV = max(min(dgradV, 20), -20);
    
    % Backstepping
    u_back = -formation_params.kp * gradV - formation_params.kd * dgradV;
    
    % Damping
    v_i = vel(:,i_drone);
    u_damp = -formation_params.beta * v_i;
    
    % =====================================================================
    %  CONNECTIVITY MAINTENANCE
    % =====================================================================
    % Tính ma trận kề sigmoid
    A = zeros(graph_params.n_drones);
    for i = 1:graph_params.n_drones
        for j = i+1:graph_params.n_drones
            d_ij = norm(pos(:,i) - pos(:,j));
            a_ij = 1 / (1 + exp(-conn_params.omega * (conn_params.d_max - d_ij)));
            A(i,j) = a_ij;
            A(j,i) = a_ij;
        end
    end
    
    % Ma trận Laplace
    D = diag(sum(A,2));
    L = D - A;
    
    % Tính M = Q'*L*Q
    Q = conn_params.Q;
    M = Q' * L * Q;
    lambda2 = min(eig(M));
    
    detM = det(M);
    if detM < 1e-6
        detM = 1e-6;
    end
    
    % Tính lực giữ liên kết bằng sai phân số
    u_conn = zeros(3, 1);
    eps_fd = 1e-4;
    
    for d = 1:graph_params.dim
        % M tại p + eps
        pos_plus = pos;
        pos_plus(d, i_drone) = pos_plus(d, i_drone) + eps_fd;
        
        A_plus = zeros(graph_params.n_drones);
        for i = 1:graph_params.n_drones
            for j = i+1:graph_params.n_drones
                d_ij = norm(pos_plus(:,i) - pos_plus(:,j));
                a_ij = 1 / (1 + exp(-conn_params.omega * (conn_params.d_max - d_ij)));
                A_plus(i,j) = a_ij;
                A_plus(j,i) = a_ij;
            end
        end
        D_plus = diag(sum(A_plus,2));
        L_plus = D_plus - A_plus;
        M_plus = Q' * L_plus * Q;
        
        % M tại p - eps
        pos_minus = pos;
        pos_minus(d, i_drone) = pos_minus(d, i_drone) - eps_fd;
        
        A_minus = zeros(graph_params.n_drones);
        for i = 1:graph_params.n_drones
            for j = i+1:graph_params.n_drones
                d_ij = norm(pos_minus(:,i) - pos_minus(:,j));
                a_ij = 1 / (1 + exp(-conn_params.omega * (conn_params.d_max - d_ij)));
                A_minus(i,j) = a_ij;
                A_minus(j,i) = a_ij;
            end
        end
        D_minus = diag(sum(A_minus,2));
        L_minus = D_minus - A_minus;
        M_minus = Q' * L_minus * Q;
        
        dM_dp = (M_plus - M_minus) / (2*eps_fd);
        
        if rcond(M) > 1e-6
            u_conn(d) = conn_params.alpha * trace(M \ dM_dp) / detM^conn_params.alpha;
        else
            u_conn(d) = 0;
        end
    end
    
    % =====================================================================
    %  OBSTACLE AVOIDANCE
    % =====================================================================
    muy = (1 + avoid_params.d_safe^4) / avoid_params.d_safe^4;
    
    % Tính beta_product
    beta_product = 1;
    for e = 1:n_edges
        i = graph_params.edges(e,1);
        j = graph_params.edges(e,2);
        dij = norm(pos(:,i) - pos(:,j));
        beta_val = beta_slide(dij, avoid_params.d_safe, muy);
        beta_product = beta_product * beta_val;
    end
    
    Phi = 1 / (beta_product^avoid_params.alpha);
    dPhi_dbeta = -avoid_params.alpha * beta_product^(-avoid_params.alpha-1);
    
    % Tính lực tránh
    u_avoid = zeros(3, 1);
    eps_deriv = 1e-4;
    
    for j = 1:graph_params.n_drones
        if j == i_drone
            continue;
        end
        
        p_ij = pos(:,i_drone) - pos(:,j);
        dij_ij = norm(p_ij);
        
        if dij_ij > 1e-6
            dd_dp = p_ij;
            
            % Đạo hàm số của beta
            beta_plus = beta_slide(dij_ij + eps_deriv, avoid_params.d_safe, muy);
            beta_minus = beta_slide(dij_ij - eps_deriv, avoid_params.d_safe, muy);
            dbeta_dd = (beta_plus - beta_minus) / (2*eps_deriv);
            
            grad = dPhi_dbeta * dbeta_dd * dd_dp;
            u_avoid = u_avoid - avoid_params.k * grad;
        end
    end
    
    u_h = [0; 0; -prior_params.k_height * (pes(3, i_drone) - pos(3, 1))];


    % =====================================================================
    %  TỔNG HỢP
    % =====================================================================
    u = 5*u_form + u_back + u_damp + 0.5*u_conn + 10*u_avoid + u_h;

end

function beta = beta_slide(dist, d_safe, muy)
    if (dist^2 - d_safe^2) >= 0
        rho = 0;
    else
        rho = 1;
    end
    diff_sq = (dist^2 - d_safe^2)^2;
    beta = (1 - muy * diff_sq / (1 + diff_sq))^rho;
    % Đảm bảo beta không âm
    beta = max(beta, 0);
end

== matlab function Ver1/Drone 3/Subsystem/Kinematic ==
  data: p_ddot output; u input
function p_ddot = fcn(u)

    p_ddot = u;

end

== matlab function Ver1/Drone 4/Subsystem/Kinematic ==
  data: p_ddot output; u input
function p_ddot = fcn(u)

    p_ddot = u;

end

== matlab function Ver1/Drone 5/MATLAB Function1 ==
  data: p input; pes input; v input; u output; params parameter Bus: params_bus
function u = fcn(p, pes, v, params)

    graph_params = params.graph_params;
    formation_params = params.formation_params;
    conn_params = params.conn_params;
    avoid_params = params.avoid_params;
    prior_params = params.prior_params;

    % Chuyển vector p thành mảng 3x5
    pos = reshape(p, 3, graph_params.n_drones);
    vel = reshape(v, 3, graph_params.n_drones);
    pes = reshape(pes, 3, graph_params.n_drones);
    
    n_edges = size(graph_params.edges, 1);
    

    i_drone = 5;
    
    % =====================================================================
    %  FORMATION CONTROL (Distance-based + Backstepping)
    % =====================================================================
    u_form = zeros(3,1);
    gradV = zeros(3,1);
    dgradV = zeros(3,1);
    
    for e = 1:n_edges
        if graph_params.edges(e,1) == i_drone
            j = graph_params.edges(e,2);
            p_ij = pos(:,j) - pos(:,i_drone);
            v_ij = vel(:,j) - vel(:,i_drone);
            dij = norm(p_ij);
            
            if dij > 1e-6
                e_ij = dij^2 - formation_params.d_star(e)^2;
                
                % Lực formation (gradient descent)
                u_form = u_form + formation_params.alpha * e_ij * p_ij;
                
                % Gradient V
                gradV = gradV + e_ij * p_ij;
                
                % Đạo hàm gradient V
                term = 2*(p_ij' * v_ij) * p_ij + e_ij * v_ij;
                dgradV = dgradV + term;
            end
            
        elseif graph_params.edges(e,2) == i_drone
            j = graph_params.edges(e,1);
            p_ij = pos(:,j) - pos(:,i_drone);
            v_ij = vel(:,j) - vel(:,i_drone);
            dij = norm(p_ij);
            
            if dij > 1e-6
                e_ij = dij^2 - formation_params.d_star(e)^2;
                
                u_form = u_form + formation_params.alpha * e_ij * p_ij;
                gradV = gradV + e_ij * p_ij;
                term = 2*(p_ij' * v_ij) * p_ij + e_ij * v_ij;
                dgradV = dgradV + term;
            end
        end
    end
    
    % Giới hạn gradient
    gradV = max(min(gradV, 15), -15);
    dgradV = max(min(dgradV, 20), -20);
    
    % Backstepping
    u_back = -formation_params.kp * gradV - formation_params.kd * dgradV;
    
    % Damping
    v_i = vel(:,i_drone);
    u_damp = -formation_params.beta * v_i;
    
    % =====================================================================
    %  CONNECTIVITY MAINTENANCE
    % =====================================================================
    % Tính ma trận kề sigmoid
    A = zeros(graph_params.n_drones);
    for i = 1:graph_params.n_drones
        for j = i+1:graph_params.n_drones
            d_ij = norm(pos(:,i) - pos(:,j));
            a_ij = 1 / (1 + exp(-conn_params.omega * (conn_params.d_max - d_ij)));
            A(i,j) = a_ij;
            A(j,i) = a_ij;
        end
    end
    
    % Ma trận Laplace
    D = diag(sum(A,2));
    L = D - A;
    
    % Tính M = Q'*L*Q
    Q = conn_params.Q;
    M = Q' * L * Q;
    lambda2 = min(eig(M));
    
    detM = det(M);
    if detM < 1e-6
        detM = 1e-6;
    end
    
    % Tính lực giữ liên kết bằng sai phân số
    u_conn = zeros(3, 1);
    eps_fd = 1e-4;
    
    for d = 1:graph_params.dim
        % M tại p + eps
        pos_plus = pos;
        pos_plus(d, i_drone) = pos_plus(d, i_drone) + eps_fd;
        
        A_plus = zeros(graph_params.n_drones);
        for i = 1:graph_params.n_drones
            for j = i+1:graph_params.n_drones
                d_ij = norm(pos_plus(:,i) - pos_plus(:,j));
                a_ij = 1 / (1 + exp(-conn_params.omega * (conn_params.d_max - d_ij)));
                A_plus(i,j) = a_ij;
                A_plus(j,i) = a_ij;
            end
        end
        D_plus = diag(sum(A_plus,2));
        L_plus = D_plus - A_plus;
        M_plus = Q' * L_plus * Q;
        
        % M tại p - eps
        pos_minus = pos;
        pos_minus(d, i_drone) = pos_minus(d, i_drone) - eps_fd;
        
        A_minus = zeros(graph_params.n_drones);
        for i = 1:graph_params.n_drones
            for j = i+1:graph_params.n_drones
                d_ij = norm(pos_minus(:,i) - pos_minus(:,j));
                a_ij = 1 / (1 + exp(-conn_params.omega * (conn_params.d_max - d_ij)));
                A_minus(i,j) = a_ij;
                A_minus(j,i) = a_ij;
            end
        end
        D_minus = diag(sum(A_minus,2));
        L_minus = D_minus - A_minus;
        M_minus = Q' * L_minus * Q;
        
        dM_dp = (M_plus - M_minus) / (2*eps_fd);
        
        if rcond(M) > 1e-6
            u_conn(d) = conn_params.alpha * trace(M \ dM_dp) / detM^conn_params.alpha;
        else
            u_conn(d) = 0;
        end
    end
    
    % =====================================================================
    %  OBSTACLE AVOIDANCE
    % =====================================================================
    muy = (1 + avoid_params.d_safe^4) / avoid_params.d_safe^4;
    
    % Tính beta_product
    beta_product = 1;
    for e = 1:n_edges
        i = graph_params.edges(e,1);
        j = graph_params.edges(e,2);
        dij = norm(pos(:,i) - pos(:,j));
        beta_val = beta_slide(dij, avoid_params.d_safe, muy);
        beta_product = beta_product * beta_val;
    end
    
    Phi = 1 / (beta_product^avoid_params.alpha);
    dPhi_dbeta = -avoid_params.alpha * beta_product^(-avoid_params.alpha-1);
    
    % Tính lực tránh
    u_avoid = zeros(3, 1);
    eps_deriv = 1e-4;
    
    for j = 1:graph_params.n_drones
        if j == i_drone
            continue;
        end
        
        p_ij = pos(:,i_drone) - pos(:,j);
        dij_ij = norm(p_ij);
        
        if dij_ij > 1e-6
            dd_dp = p_ij;
            
            % Đạo hàm số của beta
            beta_plus = beta_slide(dij_ij + eps_deriv, avoid_params.d_safe, muy);
            beta_minus = beta_slide(dij_ij - eps_deriv, avoid_params.d_safe, muy);
            dbeta_dd = (beta_plus - beta_minus) / (2*eps_deriv);
            
            grad = dPhi_dbeta * dbeta_dd * dd_dp;
            u_avoid = u_avoid - avoid_params.k * grad;
        end
    end
    
    u_h = [0; 0; -prior_params.k_height * (pes(3, i_drone) - pos(3, 1))];


    % =====================================================================
    %  TỔNG HỢP
    % =====================================================================
    u = 5*u_form + u_back + u_damp + 0.5*u_conn + 10*u_avoid + u_h;

end

function beta = beta_slide(dist, d_safe, muy)
    if (dist^2 - d_safe^2) >= 0
        rho = 0;
    else
        rho = 1;
    end
    diff_sq = (dist^2 - d_safe^2)^2;
    beta = (1 - muy * diff_sq / (1 + diff_sq))^rho;
    % Đảm bảo beta không âm
    beta = max(beta, 0);
end

== matlab function Ver1/Drone 5/Subsystem/Kinematic ==
  data: p_ddot output; u input
function p_ddot = fcn(u)

    p_ddot = u;

end

== matlab function Ver1/Virtual Trajectory/MATLAB Function ==
  data: t input; p_ref output
function p_ref = fcn(t)

    R = 50; omega = 0.2; vz = 0.5; vy = 10;

    x = R*cos(omega*t);
    y = R*sin(omega*t);

    if t < 10
        x = R*cos(omega*t);
        y = R*sin(omega*t);
        z = vz*t;
    else
        x = R*cos(omega*10);
        y = R*sin(omega*10);
        z = vz*10;
    end

    p_ref = [x; y; z];

end

== matlab function Ver1/Drone 2/Pos Estimation ==
  data: p input; v input; pes input; pes_dot output size=[3, 1]; params parameter Bus: params_bus
function pes_dot = fcn(p, v, pes, params)

    graph_params = params.graph_params;
    estimation_params = params.estimation_params;

    pes_dot = zeros(3,1);
    
    
    i_drone = 2;  % Drone đang xét
    
    % Reshape input
    pos = reshape(p, graph_params.dim, graph_params.n_drones);
    pes = reshape(pes, graph_params.dim, graph_params.n_drones);
    vel = reshape(v, graph_params.dim, graph_params.n_drones);
    
    % Tính toán gradient term
    grad_term = zeros(graph_params.dim, 1);
    
    n_edges = size(graph_params.edges, 1);
    
    for e = 1:n_edges
        if graph_params.edges(e,1) == i_drone
            j = graph_params.edges(e,2);
        else
            j = graph_params.edges(e,1);
        end

        if j == 1
            grad_term = grad_term + ((pos(:, j) - pes(:,i_drone)) - (pos(:, j) - pos(:, i_drone)));
        else
            grad_term = grad_term + (pes(:, j) - pes(:, i_drone) - (pos(:, j) - pos(:, i_drone)));
        end
    end

    
    % Output
    
    pes_dot1 = vel(:, i_drone) + estimation_params.mu*grad_term;
    pes_dot = [pes_dot1(1); pes_dot1(2); pes_dot1(3)];
end

== matlab function Ver1/Drone 3/Pos Estimation ==
  data: p input; v input; pes input; pes_dot output size=[3,1]; params parameter Bus: params_bus
function pes_dot = fcn(p, v, pes, params)

    graph_params = params.graph_params;
    estimation_params = params.estimation_params;

    pes_dot = zeros(3,1);
    
    
    i_drone = 3;  % Drone đang xét
    
    % Reshape input
    pos = reshape(p, graph_params.dim, graph_params.n_drones);
    pes = reshape(pes, graph_params.dim, graph_params.n_drones);
    vel = reshape(v, graph_params.dim, graph_params.n_drones);
    
    % Tính toán gradient term
    grad_term = zeros(graph_params.dim, 1);
    
    n_edges = size(graph_params.edges, 1);
    
    for e = 1:n_edges
        if graph_params.edges(e,1) == i_drone
            j = graph_params.edges(e,2);
        else
            j = graph_params.edges(e,1);
        end

        if j == 1
            grad_term = grad_term + ((pos(:, j) - pes(:,i_drone)) - (pos(:, j) - pos(:, i_drone)));
        else
            grad_term = grad_term + (pes(:, j) - pes(:, i_drone) - (pos(:, j) - pos(:, i_drone)));
        end
    end

    
    % Output
    
    pes_dot1 = vel(:, i_drone) + estimation_params.mu*grad_term;
    pes_dot = [pes_dot1(1); pes_dot1(2); pes_dot1(3)];
end

== matlab function Ver1/Drone 4/Pos Estimation ==
  data: p input; v input; pes input; pes_dot output size=[3,1]; params parameter Bus: params_bus
function pes_dot = fcn(p, v, pes, params)

    graph_params = params.graph_params;
    estimation_params = params.estimation_params;

    pes_dot = zeros(3,1);
    
    
    i_drone = 4;  % Drone đang xét
    
    % Reshape input
    pos = reshape(p, graph_params.dim, graph_params.n_drones);
    pes = reshape(pes, graph_params.dim, graph_params.n_drones);
    vel = reshape(v, graph_params.dim, graph_params.n_drones);
    
    % Tính toán gradient term
    grad_term = zeros(graph_params.dim, 1);
    
    n_edges = size(graph_params.edges, 1);
    
    for e = 1:n_edges
        if graph_params.edges(e,1) == i_drone
            j = graph_params.edges(e,2);
        else
            j = graph_params.edges(e,1);
        end

        if j == 1
            grad_term = grad_term + ((pos(:, j) - pes(:,i_drone)) - (pos(:, j) - pos(:, i_drone)));
        else
            grad_term = grad_term + (pes(:, j) - pes(:, i_drone) - (pos(:, j) - pos(:, i_drone)));
        end
    end

    
    % Output
    
    pes_dot1 = vel(:, i_drone) + estimation_params.mu*grad_term;
    pes_dot = [pes_dot1(1); pes_dot1(2); pes_dot1(3)];
end

== matlab function Ver1/Drone 5/Pos Estimation ==
  data: p input; v input; pes input; pes_dot output size=[3,1]; params parameter Bus: params_bus
function pes_dot = fcn(p, v, pes, params)

    graph_params = params.graph_params;
    estimation_params = params.estimation_params;

    pes_dot = zeros(3,1);
    
    
    i_drone = 5;  % Drone đang xét
    
    % Reshape input
    pos = reshape(p, graph_params.dim, graph_params.n_drones);
    pes = reshape(pes, graph_params.dim, graph_params.n_drones);
    vel = reshape(v, graph_params.dim, graph_params.n_drones);
    
    % Tính toán gradient term
    grad_term = zeros(graph_params.dim, 1);
    
    n_edges = size(graph_params.edges, 1);
    
    for e = 1:n_edges
        if graph_params.edges(e,1) == i_drone
            j = graph_params.edges(e,2);
        else
            j = graph_params.edges(e,1);
        end

        if j == 1
            grad_term = grad_term + ((pos(:, j) - pes(:,i_drone)) - (pos(:, j) - pos(:, i_drone)));
        else
            grad_term = grad_term + (pes(:, j) - pes(:, i_drone) - (pos(:, j) - pos(:, i_drone)));
        end
    end

    
    % Output
    
    pes_dot1 = vel(:, i_drone) + estimation_params.mu*grad_term;
    pes_dot = [pes_dot1(1); pes_dot1(2); pes_dot1(3)];
end
